simulink model "MCU_Stateflow_Analog"  (R2022b)
settings: Solver=FixedStepDiscrete  StartTime=0.0  StopTime=inf  FixedStep=0.002  RelTol=1e-3
undefined symbols (not defined in the file): ANALOG, cAgeingMode, cCurrentLoopMode, cNoneMode, cParaRecogMode, cSingleBoardMode, cSpeedLoopMode, cTorqueLoopMode, cVvvfOpenMode, FAULT, POWER_ON, STANDBY, TESTBED, VEHICLE, WORKING
libraries: simulink x9, SignalEditorBlockLib x1
(part 2 of 4)

== system MCU_Stateflow_Analog/Task_2ms/Arbitration/Initial ==
  note: WorkCmd初始化
  note: 在POWERON、STANDBY和FAULT模式下ModeSelect选择为cNoneMode
  Action Port : ActionPort  ActionPortLabel=if(u1 == 1)
  Constant : Constant  Value=0  OutDataTypeStr=single
  Constant1 : Constant  Value=cNoneMode  VectorParams1D=off  OutDataTypeStr=uint16
  Constant2 : Constant  Value=0  OutDataTypeStr=uint16
  Constant3 : Constant  Value=cNoneMode  VectorParams1D=off  OutDataTypeStr=uint16
  WorkState_ModeSelect : Outport
  WorkCmd_RunCmd : Outport  Port=2
  WorkCmd_DischargeCmd : Outport  Port=3
  WorkCmd_TorqueCmd : Outport  Port=4
  WorkCmd_ModeCmd : Outport  Port=5
  WorkCmd_CurrentCmd : Outport  Port=6
  WorkCmd_FreqCmd : Outport  Port=7
  WorkCmd_IsdCmd : Outport  Port=8
  WorkCmd_IsqCmd : Outport  Port=9
  WorkCmd_SpeedCmd : Outport  Port=10
  WorkCmd_ThetaCmd : Outport  Port=11
  wires:
  Constant/1 -> WorkCmd_TorqueCmd/1, WorkCmd_CurrentCmd/1, WorkCmd_FreqCmd/1, WorkCmd_ThetaCmd/1, WorkCmd_SpeedCmd/1, WorkCmd_IsqCmd/1, WorkCmd_IsdCmd/1
  Constant1/1 -> WorkState_ModeSelect/1
  Constant2/1 -> WorkCmd_RunCmd/1, WorkCmd_DischargeCmd/1
  Constant3/1 -> WorkCmd_ModeCmd/1

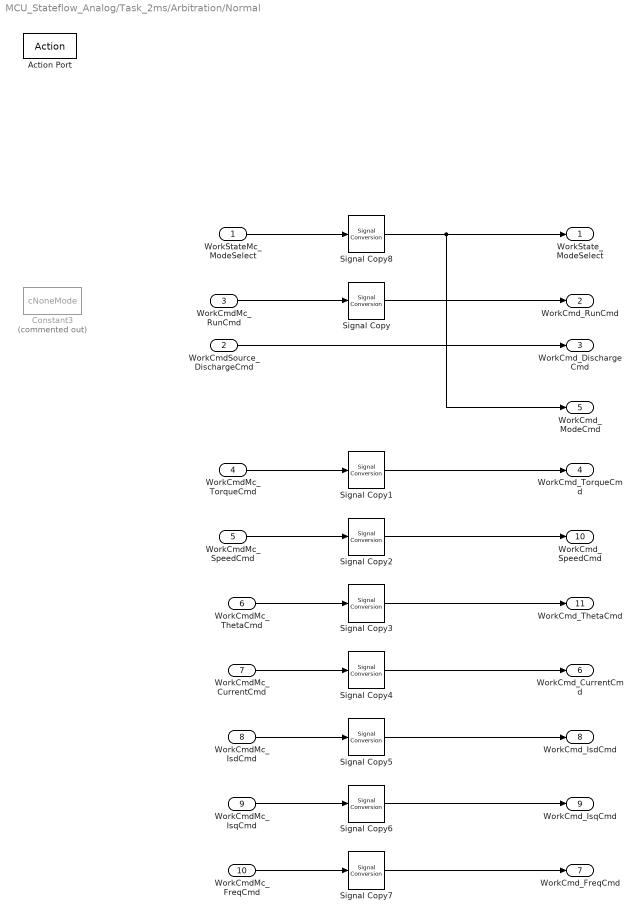
== system MCU_Stateflow_Analog/Task_2ms/Arbitration/Normal ==
  WorkStateMc_ModeSelect : Inport
  WorkCmdSource_DischargeCmd : Inport  Port=2
  WorkCmdMc_RunCmd : Inport  Port=3
  WorkCmdMc_TorqueCmd : Inport  Port=4
  WorkCmdMc_SpeedCmd : Inport  Port=5
  WorkCmdMc_ThetaCmd : Inport  Port=6
  WorkCmdMc_CurrentCmd : Inport  Port=7
  WorkCmdMc_IsdCmd : Inport  Port=8
  WorkCmdMc_IsqCmd : Inport  Port=9
  WorkCmdMc_FreqCmd : Inport  Port=10
  Action Port : ActionPort  ActionPortLabel=else
  Constant3 : Constant  Commented=on  Value=cNoneMode  VectorParams1D=off  OutDataTypeStr=uint16
  Signal Copy{,1..8} (9 alike) : SignalConversion  OverrideOpt=off
  WorkState_ModeSelect : Outport
  WorkCmd_RunCmd : Outport  Port=2
  WorkCmd_DischargeCmd : Outport  Port=3
  WorkCmd_TorqueCmd : Outport  Port=4
  WorkCmd_ModeCmd : Outport  Port=5
  WorkCmd_CurrentCmd : Outport  Port=6
  WorkCmd_FreqCmd : Outport  Port=7
  WorkCmd_IsdCmd : Outport  Port=8
  WorkCmd_IsqCmd : Outport  Port=9
  WorkCmd_SpeedCmd : Outport  Port=10
  WorkCmd_ThetaCmd : Outport  Port=11
  wires:
  WorkCmdMc_RunCmd/1 -> Signal Copy/1
  WorkCmdMc_TorqueCmd/1 -> Signal Copy1/1
  WorkCmdMc_SpeedCmd/1 -> Signal Copy2/1
  WorkCmdMc_ThetaCmd/1 -> Signal Copy3/1
  WorkCmdMc_CurrentCmd/1 -> Signal Copy4/1
  WorkCmdMc_IsdCmd/1 -> Signal Copy5/1
  WorkCmdMc_IsqCmd/1 -> Signal Copy6/1
  WorkCmdMc_FreqCmd/1 -> Signal Copy7/1
  WorkStateMc_ModeSelect/1 -> Signal Copy8/1
  Signal Copy8/1 -> WorkCmd_ModeCmd/1, WorkState_ModeSelect/1
  Signal Copy/1 -> WorkCmd_RunCmd/1
  Signal Copy1/1 -> WorkCmd_TorqueCmd/1
  Signal Copy2/1 -> WorkCmd_SpeedCmd/1
  Signal Copy3/1 -> WorkCmd_ThetaCmd/1
  Signal Copy4/1 -> WorkCmd_CurrentCmd/1
  Signal Copy5/1 -> WorkCmd_IsdCmd/1
  Signal Copy6/1 -> WorkCmd_IsqCmd/1
  Signal Copy7/1 -> WorkCmd_FreqCmd/1
  WorkCmdSource_DischargeCmd/1 -> WorkCmd_DischargeCmd/1

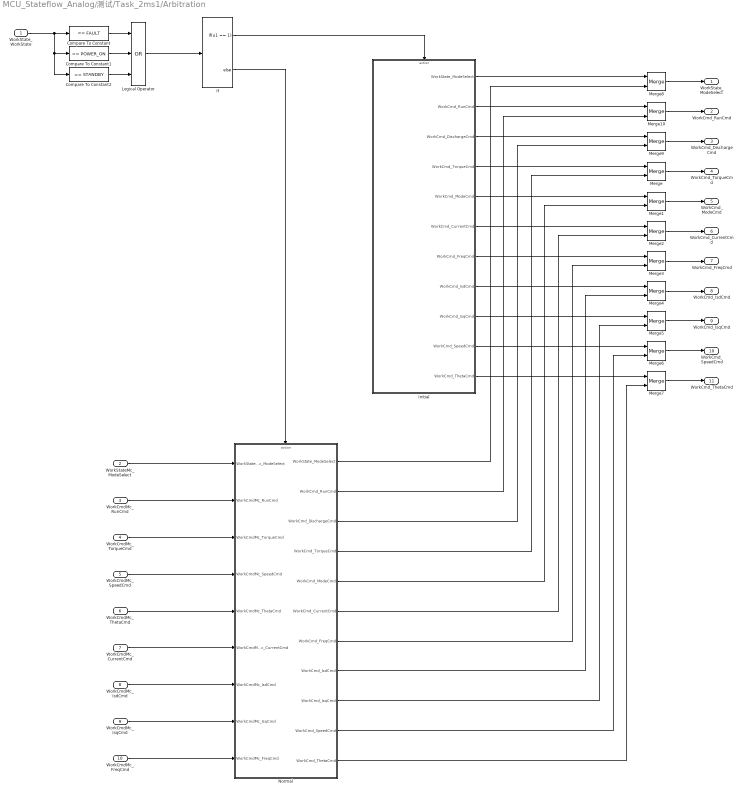
== system MCU_Stateflow_Analog/测试/Task_2ms1/Arbitration ==
  WorkState_WorkState : Inport
  WorkStateMc_ModeSelect : Inport  Port=2
  WorkCmdMc_RunCmd : Inport  Port=3
  WorkCmdMc_TorqueCmd : Inport  Port=4
  WorkCmdMc_SpeedCmd : Inport  Port=5
  WorkCmdMc_ThetaCmd : Inport  Port=6
  WorkCmdMc_CurrentCmd : Inport  Port=7
  WorkCmdMc_IsdCmd : Inport  Port=8
  WorkCmdMc_IsqCmd : Inport  Port=9
  WorkCmdMc_FreqCmd : Inport  Port=10
  Compare To Constant : simulink/Logic and Bit Operations/Compare To Constant  relop===  const=FAULT  OutDataTypeStr=boolean
  Compare To Constant1 : simulink/Logic and Bit Operations/Compare To Constant  relop===  const=POWER_ON  OutDataTypeStr=boolean
  Compare To Constant2 : simulink/Logic and Bit Operations/Compare To Constant  relop===  const=STANDBY  OutDataTypeStr=boolean
  If : If  IfExpression=u1 == 1
  Initial : Subsystem  TreatAsAtomicUnit=on
  Logical Operator : Logic  Operator=OR  Inputs=3  AllPortsSameDT=off  OutDataTypeStr=boolean
  Merge{,1..10} (11 alike) : Merge
  Normal : Subsystem  TreatAsAtomicUnit=on
  WorkState_ModeSelect : Outport
  WorkCmd_RunCmd : Outport  Port=2
  WorkCmd_DischargeCmd : Outport  Port=3
  WorkCmd_TorqueCmd : Outport  Port=4
  WorkCmd_ModeCmd : Outport  Port=5
  WorkCmd_CurrentCmd : Outport  Port=6
  WorkCmd_FreqCmd : Outport  Port=7
  WorkCmd_IsdCmd : Outport  Port=8
  WorkCmd_IsqCmd : Outport  Port=9
  WorkCmd_SpeedCmd : Outport  Port=10
  WorkCmd_ThetaCmd : Outport  Port=11
  wires:
  WorkState_WorkState/1 -> Compare To Constant2/1, Compare To Constant1/1, Compare To Constant/1
  Compare To Constant/1 -> Logical Operator/1
  Compare To Constant1/1 -> Logical Operator/2
  Compare To Constant2/1 -> Logical Operator/3
  Logical Operator/1 -> If/1
  If/1 -> Initial/Action
  If/2 -> Normal/Action
  Initial/11(WorkCmd_ThetaCmd) -> Merge7/1
  Initial/10(WorkCmd_SpeedCmd) -> Merge6/1
  Initial/9(WorkCmd_IsqCmd) -> Merge5/1
  Initial/8(WorkCmd_IsdCmd) -> Merge4/1
  Initial/7(WorkCmd_FreqCmd) -> Merge3/1
  Initial/6(WorkCmd_CurrentCmd) -> Merge2/1
  Initial/5(WorkCmd_ModeCmd) -> Merge1/1
  Initial/4(WorkCmd_TorqueCmd) -> Merge/1
  Initial/3(WorkCmd_DischargeCmd) -> Merge9/1
  WorkStateMc_ModeSelect/1 -> Normal/1(WorkStateMc_ModeSelect)
  WorkCmdMc_RunCmd/1 -> Normal/2(WorkCmdMc_RunCmd)
  WorkCmdMc_TorqueCmd/1 -> Normal/3(WorkCmdMc_TorqueCmd)
  WorkCmdMc_SpeedCmd/1 -> Normal/4(WorkCmdMc_SpeedCmd)
  WorkCmdMc_ThetaCmd/1 -> Normal/5(WorkCmdMc_ThetaCmd)
  WorkCmdMc_CurrentCmd/1 -> Normal/6(WorkCmdMc_CurrentCmd)
  WorkCmdMc_IsdCmd/1 -> Normal/7(WorkCmdMc_IsdCmd)
  WorkCmdMc_IsqCmd/1 -> Normal/8(WorkCmdMc_IsqCmd)
  WorkCmdMc_FreqCmd/1 -> Normal/9(WorkCmdMc_FreqCmd)
  Merge/1 -> WorkCmd_TorqueCmd/1
  Merge1/1 -> WorkCmd_ModeCmd/1
  Merge2/1 -> WorkCmd_CurrentCmd/1
  Merge3/1 -> WorkCmd_FreqCmd/1
  Merge4/1 -> WorkCmd_IsdCmd/1
  Merge5/1 -> WorkCmd_IsqCmd/1
  Merge6/1 -> WorkCmd_SpeedCmd/1
  Merge7/1 -> WorkCmd_ThetaCmd/1
  Initial/1(WorkState_ModeSelect) -> Merge8/1
  Merge8/1 -> WorkState_ModeSelect/1
  Initial/2(WorkCmd_RunCmd) -> Merge10/1
  Merge10/1 -> WorkCmd_RunCmd/1
  Merge9/1 -> WorkCmd_DischargeCmd/1
  Normal/1(WorkState_ModeSelect) -> Merge8/2
  Normal/2(WorkCmd_RunCmd) -> Merge10/2
  Normal/3(WorkCmd_DischargeCmd) -> Merge9/2
  Normal/4(WorkCmd_TorqueCmd) -> Merge/2
  Normal/5(WorkCmd_ModeCmd) -> Merge1/2
  Normal/6(WorkCmd_CurrentCmd) -> Merge2/2
  Normal/7(WorkCmd_FreqCmd) -> Merge3/2
  Normal/8(WorkCmd_IsdCmd) -> Merge4/2
  Normal/9(WorkCmd_IsqCmd) -> Merge5/2
  Normal/10(WorkCmd_SpeedCmd) -> Merge6/2
  Normal/11(WorkCmd_ThetaCmd) -> Merge7/2

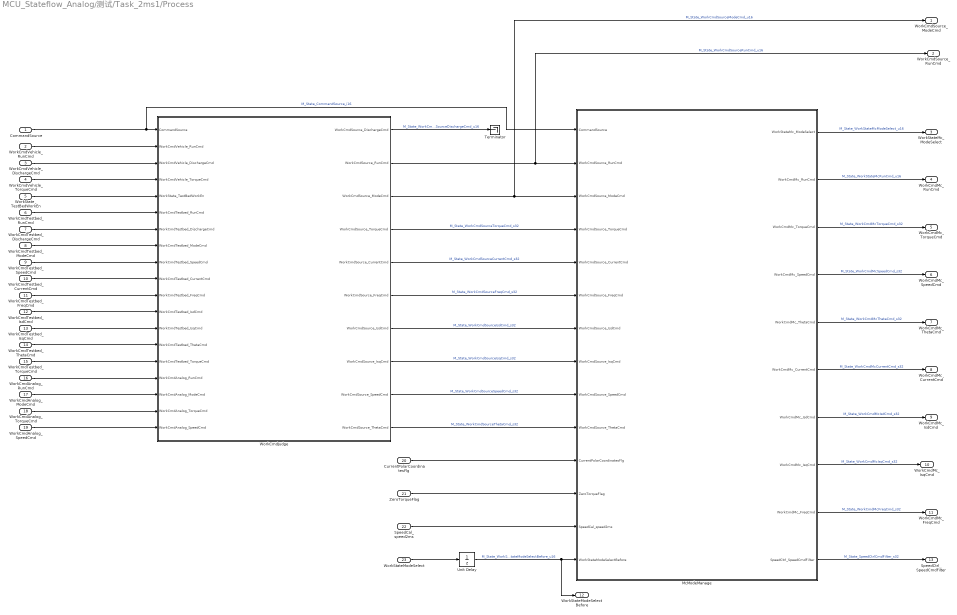
== system MCU_Stateflow_Analog/测试/Task_2ms1/Process ==
  CommandSource : Inport
  WorkCmdVehicle_RunCmd : Inport  Port=2
  WorkCmdVehicle_DischargeCmd : Inport  Port=3
  WorkCmdVehicle_TorqueCmd : Inport  Port=4
  WorkState_TestBedWorkEn : Inport  Port=5
  WorkCmdTestbed_RunCmd : Inport  Port=6
  WorkCmdTestbed_DischargeCmd : Inport  Port=7
  WorkCmdTestbed_ModeCmd : Inport  Port=8
  WorkCmdTestbed_SpeedCmd : Inport  Port=9
  WorkCmdTestbed_CurrentCmd : Inport  Port=10
  WorkCmdTestbed_FreqCmd : Inport  Port=11
  WorkCmdTestbed_IsdCmd : Inport  Port=12
  WorkCmdTestbed_IsqCmd : Inport  Port=13
  WorkCmdTestbed_ThetaCmd : Inport  Port=14
  WorkCmdTestbed_TorqueCmd : Inport  Port=15
  WorkCmdAnalog_RunCmd : Inport  Port=16
  WorkCmdAnalog_ModeCmd : Inport  Port=17
  WorkCmdAnalog_TorqueCmd : Inport  Port=18
  WorkCmdAnalog_SpeedCmd : Inport  Port=19
  CurrentPolarCoordinatesFlg : Inport  Port=20
  ZeroTorqueFlag : Inport  Port=21
  SpeedCal_speed2ms : Inport  Port=22
  WorkStateModeSelect : Inport  Port=23
  McModeManage : Stateflow chart  TreatAsAtomicUnit=on
      settings: RTWSystemCode=Nonreusable function  PortSchema="{\"entries\":[{\"content\":{\"sides\":[{\"content\":{\"connectorIds\":[\"In2\",\"In4\",\"In3\",\"In5\",\"In6\",\"In7\",\"In8\",\"In9\",\"In10\",\"In1\",\"In11\",\"In12\",\"In13\",\"In14\"]},\"type\":\"ConnectorPlacement.EquallySpacedRectSide\",\"uuid\":\"2e7d3842-0a61-4590-9292-7a5bc1b6d63e\"},{\"content\":{\"connectorIds\":[\"Out1\",\"Out2\",\"Out3\",\"Out4\",\"Out5\",\"Out6\",\"Out7\",\"Out8\",\"Out9\",\"Out10\"],\"side\":\"RIGHT\"},\"type\":\"ConnectorPlacement.EquallySpacedRectSide\",\"uuid\":\"fb66f02a-321f-47a6-a489-4b94442e22c8\"},{\"content\":{\"connectorIds\":[],\"side\":\"TOP\"},\"type\":\"ConnectorPlacement.EquallySpacedRectSide\",\"uuid\":\"26cfdcf8-827e-48d9-aa42-40739db869be\"},{\"content\":{\"connectorIds\":[],\"side\":\"BOTTOM\"},\"type\":\"ConnectorPlacement.EquallySpacedRectSide\",\"uuid\":\"3bc2be8d-756f-48d1-976e-919451ea6fa2\"}]},\"type\":\"ConnectorPlacement.EquallySpacedConnector\",\"uuid\":\"eb156a25-beb1-4594-a414-e9203ec852c3\"}],\"packageUris\":[\"http://schema.mathworks.com/mf0/Connector/R2020b\"],\"version\":\"1.0\"}"
  Terminator : Terminator
  Unit Delay : UnitDelay  SampleTime=-1  HasFrameUpgradeWarning=on
  WorkCmdJudge : Stateflow chart  TreatAsAtomicUnit=on
      settings: RTWSystemCode=Nonreusable function  PortSchema="{\"entries\":[{\"content\":{\"sides\":[{\"content\":{\"connectorIds\":[\"In2\",\"In3\",\"In4\",\"In15\",\"In5\",\"In6\",\"In7\",\"In8\",\"In9\",\"In10\",\"In11\",\"In12\",\"In13\",\"In14\",\"In16\",\"In17\",\"In1\",\"In19\",\"In18\"]},\"type\":\"ConnectorPlacement.EquallySpacedRectSide\",\"uuid\":\"08f79912-2405-4f04-9254-689ee53f44b9\"},{\"content\":{\"connectorIds\":[\"Out1\",\"Out2\",\"Out3\",\"Out10\",\"Out4\",\"Out5\",\"Out6\",\"Out7\",\"Out8\",\"Out9\"],\"side\":\"RIGHT\"},\"type\":\"ConnectorPlacement.EquallySpacedRectSide\",\"uuid\":\"8406ee0b-fe03-429b-8d11-a315759dccf9\"},{\"content\":{\"connectorIds\":[],\"side\":\"TOP\"},\"type\":\"ConnectorPlacement.EquallySpacedRectSide\",\"uuid\":\"82a87416-6ee6-4a7e-925f-181c5fe86ae8\"},{\"content\":{\"connectorIds\":[],\"side\":\"BOTTOM\"},\"type\":\"ConnectorPlacement.EquallySpacedRectSide\",\"uuid\":\"850ffd8e-4d4e-428c-999d-6858cee77358\"}]},\"type\":\"ConnectorPlacement.EquallySpacedConnector\",\"uuid\":\"ba5e9ad6-4f64-4c0c-82e6-bf977e3fd6e6\"}],\"packageUris\":[\"http://schema.mathworks.com/mf0/Connector/R2020b\"],\"version\":\"1.0\"}"
  WorkCmdSource_ModeCmd : Outport
  WorkCmdSource_RunCmd : Outport  Port=2
  WorkStateMc_ModeSelect : Outport  Port=3
  WorkCmdMc_RunCmd : Outport  Port=4
  WorkCmdMc_TorqueCmd : Outport  Port=5
  WorkCmdMc_SpeedCmd : Outport  Port=6
  WorkCmdMc_ThetaCmd : Outport  Port=7
  WorkCmdMc_CurrentCmd : Outport  Port=8
  WorkCmdMc_IsdCmd : Outport  Port=9
  WorkCmdMc_IsqCmd : Outport  Port=10
  WorkCmdMc_FreqCmd : Outport  Port=11
  WorkStateModeSelectBefore : Outport  Port=12
  SpeedCtrl_SpeedCmdFilter : Outport  Port=13
  wires:
  WorkCmdJudge/8(WorkCmdSource_SpeedCmd) -> McModeManage/10(WorkCmdSource_SpeedCmd)  "M_State_WorkCmdSourceSpeedCmd_s32"
  CommandSource/1 -> WorkCmdJudge/2(CommandSource), McModeManage/2(CommandSource)  "M_State_CommandSource_i16"
  WorkCmdJudge/4(WorkCmdSource_CurrentCmd) -> McModeManage/6(WorkCmdSource_CurrentCmd)  "M_State_WorkCmdSourceCurrentCmd_s32"
  WorkCmdJudge/6(WorkCmdSource_IsdCmd) -> McModeManage/8(WorkCmdSource_IsdCmd)  "M_State_WorkCmdSourceIsdCmd_s32"
  WorkCmdJudge/2(WorkCmdSource_RunCmd) -> WorkCmdSource_RunCmd/1, McModeManage/4(WorkCmdSource_RunCmd)  "M_State_WorkCmdSourceRunCmd_u16"
  WorkCmdTestbed_ThetaCmd/1 -> WorkCmdJudge/14(WorkCmdTestbed_ThetaCmd)
  WorkCmdJudge/7(WorkCmdSource_IsqCmd) -> McModeManage/9(WorkCmdSource_IsqCmd)  "M_State_WorkCmdSourceIsqCmd_s32"
  McModeManage/9(WorkCmdMc_FreqCmd) -> WorkCmdMc_FreqCmd/1  "M_State_WorkCmdMcFreqCmd_s32"
  McModeManage/2(WorkCmdMc_RunCmd) -> WorkCmdMc_RunCmd/1  "M_State_WorkStateMcRunCmd_u16"
  WorkCmdJudge/5(WorkCmdSource_FreqCmd) -> McModeManage/7(WorkCmdSource_FreqCmd)  "M_State_WorkCmdSourceFreqCmd_s32"
  WorkCmdJudge/10(WorkCmdSource_TorqueCmd) -> McModeManage/5(WorkCmdSource_TorqueCmd)  "M_State_WorkCmdSourceTorqueCmd_s32"
  McModeManage/4(WorkCmdMc_SpeedCmd) -> WorkCmdMc_SpeedCmd/1  "M_State_WorkCmdMcSpeedCmd_s32"
  WorkCmdJudge/9(WorkCmdSource_ThetaCmd) -> McModeManage/1(WorkCmdSource_ThetaCmd)  "M_State_WorkCmdSourceThetaCmd_s32"
  WorkCmdVehicle_RunCmd/1 -> WorkCmdJudge/3(WorkCmdVehicle_RunCmd)
  WorkCmdTestbed_IsdCmd/1 -> WorkCmdJudge/12(WorkCmdTestbed_IsdCmd)
  WorkCmdTestbed_IsqCmd/1 -> WorkCmdJudge/13(WorkCmdTestbed_IsqCmd)
  WorkCmdJudge/1(WorkCmdSource_DischargeCmd) -> Terminator/1  "M_State_WorkCmdSourceDischargeCmd_u16"
  McModeManage/1(WorkStateMc_ModeSelect) -> WorkStateMc_ModeSelect/1  "M_State_WorkStateMcModeSelect_u16"
  WorkCmdTestbed_TorqueCmd/1 -> WorkCmdJudge/16(WorkCmdTestbed_TorqueCmd)
  WorkCmdJudge/3(WorkCmdSource_ModeCmd) -> WorkCmdSource_ModeCmd/1, McModeManage/3(WorkCmdSource_ModeCmd)  "M_State_WorkCmdSourceModeCmd_u16"
  WorkCmdTestbed_ModeCmd/1 -> WorkCmdJudge/8(WorkCmdTestbed_ModeCmd)
  WorkCmdTestbed_DischargeCmd/1 -> WorkCmdJudge/7(WorkCmdTestbed_DischargeCmd)
  WorkCmdTestbed_RunCmd/1 -> WorkCmdJudge/6(WorkCmdTestbed_RunCmd)
  WorkCmdVehicle_DischargeCmd/1 -> WorkCmdJudge/4(WorkCmdVehicle_DischargeCmd)
  WorkCmdVehicle_TorqueCmd/1 -> WorkCmdJudge/15(WorkCmdVehicle_TorqueCmd)
  WorkState_TestBedWorkEn/1 -> WorkCmdJudge/5(WorkState_TestBedWorkEn)
  WorkCmdTestbed_CurrentCmd/1 -> WorkCmdJudge/10(WorkCmdTestbed_CurrentCmd)
  McModeManage/6(WorkCmdMc_CurrentCmd) -> WorkCmdMc_CurrentCmd/1  "M_State_WorkCmdMcCurrentCmd_s32"
  McModeManage/5(WorkCmdMc_ThetaCmd) -> WorkCmdMc_ThetaCmd/1  "M_State_WorkCmdMcThetaCmd_s32"
  McModeManage/7(WorkCmdMc_IsdCmd) -> WorkCmdMc_IsdCmd/1  "M_State_WorkCmdMcIsdCmd_s32"
  WorkCmdTestbed_SpeedCmd/1 -> WorkCmdJudge/9(WorkCmdTestbed_SpeedCmd)
  McModeManage/3(WorkCmdMc_TorqueCmd) -> WorkCmdMc_TorqueCmd/1  "M_State_WorkCmdMcTorqueCmd_s32"
  McModeManage/8(WorkCmdMc_IsqCmd) -> WorkCmdMc_IsqCmd/1  "M_State_WorkCmdMcIsqCmd_s32"
  WorkCmdTestbed_FreqCmd/1 -> WorkCmdJudge/11(WorkCmdTestbed_FreqCmd)
  WorkStateModeSelect/1 -> Unit Delay/1
  Unit Delay/1 -> McModeManage/14(WorkStateModeSelectBefore), WorkStateModeSelectBefore/1  "M_State_WorkStateModeSelectBefore_u16"
  WorkCmdAnalog_RunCmd/1 -> WorkCmdJudge/17(WorkCmdAnalog_RunCmd)
  WorkCmdAnalog_ModeCmd/1 -> WorkCmdJudge/1(WorkCmdAnalog_ModeCmd)
  WorkCmdAnalog_TorqueCmd/1 -> WorkCmdJudge/19(WorkCmdAnalog_TorqueCmd)
  WorkCmdAnalog_SpeedCmd/1 -> WorkCmdJudge/18(WorkCmdAnalog_SpeedCmd)
  CurrentPolarCoordinatesFlg/1 -> McModeManage/11(CurrentPolarCoordinatesFlg)
  ZeroTorqueFlag/1 -> McModeManage/12(ZeroTorqueFlag)
  SpeedCal_speed2ms/1 -> McModeManage/13(SpeedCal_speed2ms)
  McModeManage/10(SpeedCtrl_SpeedCmdFilter) -> SpeedCtrl_SpeedCmdFilter/1  "M_State_SpeedCtrlCmdFilter_s32"

== system MCU_Stateflow_Analog/测试/Task_2ms1/草稿 ==
  Chart : Stateflow chart  Commented=on  TreatAsAtomicUnit=on
      settings: PortSchema="{\"entries\":[{\"content\":{\"sides\":[{\"content\":{\"connectorIds\":[\"In2\",\"In4\",\"In3\",\"In5\",\"In6\",\"In7\",\"In8\",\"In9\",\"In10\",\"In11\",\"In1\"]},\"type\":\"ConnectorPlacement.EquallySpacedRectSide\",\"uuid\":\"2e7d3842-0a61-4590-9292-7a5bc1b6d63e\"},{\"content\":{\"connectorIds\":[\"Out1\",\"Out2\",\"Out3\",\"Out4\",\"Out5\",\"Out6\",\"Out7\",\"Out8\",\"Out9\"],\"side\":\"RIGHT\"},\"type\":\"ConnectorPlacement.EquallySpacedRectSide\",\"uuid\":\"fb66f02a-321f-47a6-a489-4b94442e22c8\"},{\"content\":{\"connectorIds\":[],\"side\":\"TOP\"},\"type\":\"ConnectorPlacement.EquallySpacedRectSide\",\"uuid\":\"26cfdcf8-827e-48d9-aa42-40739db869be\"},{\"content\":{\"connectorIds\":[],\"side\":\"BOTTOM\"},\"type\":\"ConnectorPlacement.EquallySpacedRectSide\",\"uuid\":\"3bc2be8d-756f-48d1-976e-919451ea6fa2\"}]},\"type\":\"ConnectorPlacement.EquallySpacedConnector\",\"uuid\":\"eb156a25-beb1-4594-a414-e9203ec852c3\"}],\"packageUris\":[\"http://schema.mathworks.com/mf0/Connector/R2020b\"],\"version\":\"1.0\"}"
  Chart2 : Stateflow chart  Commented=on  TreatAsAtomicUnit=on
      settings: PortSchema="{\"entries\":[{\"content\":{\"sides\":[{\"content\":{\"connectorIds\":[\"In2\",\"In4\",\"In3\",\"In5\",\"In6\",\"In7\",\"In8\",\"In9\",\"In10\",\"In1\",\"In11\"]},\"type\":\"ConnectorPlacement.EquallySpacedRectSide\",\"uuid\":\"2e7d3842-0a61-4590-9292-7a5bc1b6d63e\"},{\"content\":{\"connectorIds\":[\"Out1\",\"Out2\",\"Out3\",\"Out4\",\"Out5\",\"Out6\",\"Out7\",\"Out8\",\"Out9\"],\"side\":\"RIGHT\"},\"type\":\"ConnectorPlacement.EquallySpacedRectSide\",\"uuid\":\"fb66f02a-321f-47a6-a489-4b94442e22c8\"},{\"content\":{\"connectorIds\":[],\"side\":\"TOP\"},\"type\":\"ConnectorPlacement.EquallySpacedRectSide\",\"uuid\":\"26cfdcf8-827e-48d9-aa42-40739db869be\"},{\"content\":{\"connectorIds\":[],\"side\":\"BOTTOM\"},\"type\":\"ConnectorPlacement.EquallySpacedRectSide\",\"uuid\":\"3bc2be8d-756f-48d1-976e-919451ea6fa2\"}]},\"type\":\"ConnectorPlacement.EquallySpacedConnector\",\"uuid\":\"eb156a25-beb1-4594-a414-e9203ec852c3\"}],\"packageUris\":[\"http://schema.mathworks.com/mf0/Connector/R2020b\"],\"version\":\"1.0\"}"
  MotorState1 : Stateflow chart  Commented=on  TreatAsAtomicUnit=on
  MotorState2 : Stateflow chart  Commented=on  TreatAsAtomicUnit=on
      settings: PortSchema="{\"entries\":[{\"content\":{\"sides\":[{\"content\":{\"connectorIds\":[\"In12\",\"In7\",\"In8\",\"In9\",\"In10\",\"In11\",\"In13\",\"In14\",\"In6\",\"In15\",\"In5\",\"In4\",\"In3\",\"In2\",\"In1\"]},\"type\":\"ConnectorPlacement.EquallySpacedRectSide\",\"uuid\":\"e0adab7d-9c82-44fd-b38c-331bb9d71454\"},{\"content\":{\"connectorIds\":[\"Out1\",\"Out2\",\"Out3\"],\"side\":\"RIGHT\"},\"type\":\"ConnectorPlacement.EquallySpacedRectSide\",\"uuid\":\"98ad1acc-debf-46f0-91aa-4bd2062f60b6\"},{\"content\":{\"connectorIds\":[],\"side\":\"TOP\"},\"type\":\"ConnectorPlacement.EquallySpacedRectSide\",\"uuid\":\"a7c2d312-245c-4ce1-bea5-1bac95c515f1\"},{\"content\":{\"connectorIds\":[],\"side\":\"BOTTOM\"},\"type\":\"ConnectorPlacement.EquallySpacedRectSide\",\"uuid\":\"175f3b6b-1019-4e6e-83d9-bf4c82f74bc8\"}]},\"type\":\"ConnectorPlacement.EquallySpacedConnector\",\"uuid\":\"df312d8c-c57e-4b1a-958b-330641c1b4d1\"}],\"packageUris\":[\"http://schema.mathworks.com/mf0/Connector/R2020b\"],\"version\":\"1.0\"}"
  MotorState3 : Stateflow chart  TreatAsAtomicUnit=on
      settings: PortSchema="{\"entries\":[{\"content\":{\"sides\":[{\"content\":{\"connectorIds\":[\"In5\",\"In1\",\"In2\",\"In3\",\"In4\"]},\"type\":\"ConnectorPlacement.EquallySpacedRectSide\",\"uuid\":\"e0adab7d-9c82-44fd-b38c-331bb9d71454\"},{\"content\":{\"connectorIds\":[\"Out1\",\"Out2\",\"Out3\"],\"side\":\"RIGHT\"},\"type\":\"ConnectorPlacement.EquallySpacedRectSide\",\"uuid\":\"98ad1acc-debf-46f0-91aa-4bd2062f60b6\"},{\"content\":{\"connectorIds\":[],\"side\":\"TOP\"},\"type\":\"ConnectorPlacement.EquallySpacedRectSide\",\"uuid\":\"a7c2d312-245c-4ce1-bea5-1bac95c515f1\"},{\"content\":{\"connectorIds\":[],\"side\":\"BOTTOM\"},\"type\":\"ConnectorPlacement.EquallySpacedRectSide\",\"uuid\":\"175f3b6b-1019-4e6e-83d9-bf4c82f74bc8\"}]},\"type\":\"ConnectorPlacement.EquallySpacedConnector\",\"uuid\":\"df312d8c-c57e-4b1a-958b-330641c1b4d1\"}],\"packageUris\":[\"http://schema.mathworks.com/mf0/Connector/R2020b\"],\"version\":\"1.0\"}"
  MotorState4 : Stateflow chart  Commented=on  TreatAsAtomicUnit=on
      settings: PortSchema="{\"entries\":[{\"content\":{\"sides\":[{\"content\":{\"connectorIds\":[\"In4\",\"In3\",\"In1\",\"In2\",\"In5\"]},\"type\":\"ConnectorPlacement.EquallySpacedRectSide\",\"uuid\":\"e0adab7d-9c82-44fd-b38c-331bb9d71454\"},{\"content\":{\"connectorIds\":[\"Out1\",\"Out2\",\"Out3\"],\"side\":\"RIGHT\"},\"type\":\"ConnectorPlacement.EquallySpacedRectSide\",\"uuid\":\"98ad1acc-debf-46f0-91aa-4bd2062f60b6\"},{\"content\":{\"connectorIds\":[],\"side\":\"TOP\"},\"type\":\"ConnectorPlacement.EquallySpacedRectSide\",\"uuid\":\"a7c2d312-245c-4ce1-bea5-1bac95c515f1\"},{\"content\":{\"connectorIds\":[],\"side\":\"BOTTOM\"},\"type\":\"ConnectorPlacement.EquallySpacedRectSide\",\"uuid\":\"175f3b6b-1019-4e6e-83d9-bf4c82f74bc8\"}]},\"type\":\"ConnectorPlacement.EquallySpacedConnector\",\"uuid\":\"df312d8c-c57e-4b1a-958b-330641c1b4d1\"}],\"packageUris\":[\"http://schema.mathworks.com/mf0/Connector/R2020b\"],\"version\":\"1.0\"}"

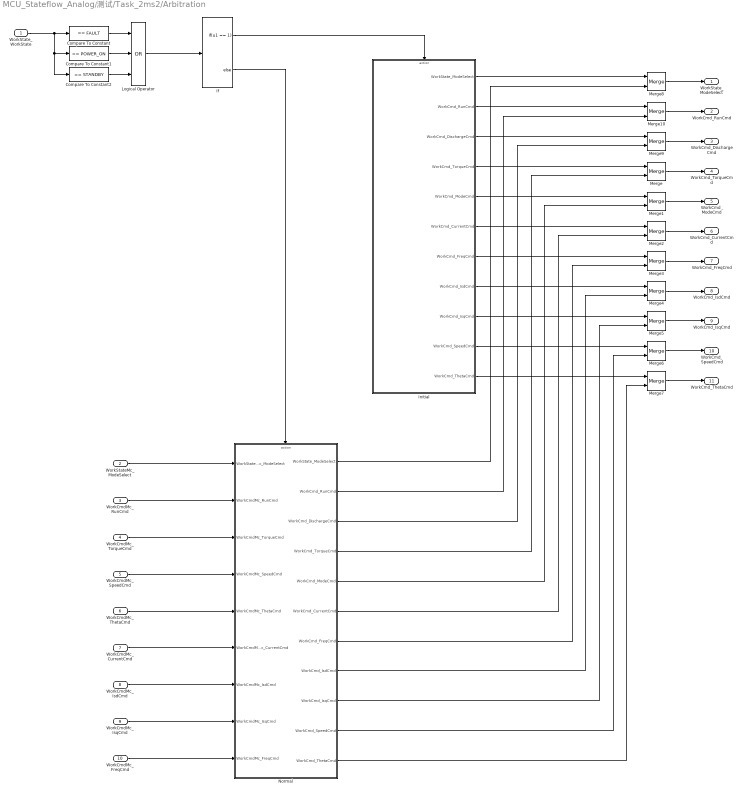
== system MCU_Stateflow_Analog/测试/Task_2ms2/Arbitration ==
  WorkState_WorkState : Inport
  WorkStateMc_ModeSelect : Inport  Port=2
  WorkCmdMc_RunCmd : Inport  Port=3
  WorkCmdMc_TorqueCmd : Inport  Port=4
  WorkCmdMc_SpeedCmd : Inport  Port=5
  WorkCmdMc_ThetaCmd : Inport  Port=6
  WorkCmdMc_CurrentCmd : Inport  Port=7
  WorkCmdMc_IsdCmd : Inport  Port=8
  WorkCmdMc_IsqCmd : Inport  Port=9
  WorkCmdMc_FreqCmd : Inport  Port=10
  Compare To Constant : simulink/Logic and Bit Operations/Compare To Constant  relop===  const=FAULT  OutDataTypeStr=boolean
  Compare To Constant1 : simulink/Logic and Bit Operations/Compare To Constant  relop===  const=POWER_ON  OutDataTypeStr=boolean
  Compare To Constant2 : simulink/Logic and Bit Operations/Compare To Constant  relop===  const=STANDBY  OutDataTypeStr=boolean
  If : If  IfExpression=u1 == 1
  Initial : Subsystem  TreatAsAtomicUnit=on
  Logical Operator : Logic  Operator=OR  Inputs=3  AllPortsSameDT=off  OutDataTypeStr=boolean
  Merge{,1..10} (11 alike) : Merge
  Normal : Subsystem  TreatAsAtomicUnit=on
  WorkState_ModeSelect : Outport
  WorkCmd_RunCmd : Outport  Port=2
  WorkCmd_DischargeCmd : Outport  Port=3
  WorkCmd_TorqueCmd : Outport  Port=4
  WorkCmd_ModeCmd : Outport  Port=5
  WorkCmd_CurrentCmd : Outport  Port=6
  WorkCmd_FreqCmd : Outport  Port=7
  WorkCmd_IsdCmd : Outport  Port=8
  WorkCmd_IsqCmd : Outport  Port=9
  WorkCmd_SpeedCmd : Outport  Port=10
  WorkCmd_ThetaCmd : Outport  Port=11
  wires:
  WorkState_WorkState/1 -> Compare To Constant2/1, Compare To Constant1/1, Compare To Constant/1
  Compare To Constant/1 -> Logical Operator/1
  Compare To Constant1/1 -> Logical Operator/2
  Compare To Constant2/1 -> Logical Operator/3
  Logical Operator/1 -> If/1
  If/1 -> Initial/Action
  If/2 -> Normal/Action
  Initial/11(WorkCmd_ThetaCmd) -> Merge7/1
  Initial/10(WorkCmd_SpeedCmd) -> Merge6/1
  Initial/9(WorkCmd_IsqCmd) -> Merge5/1
  Initial/8(WorkCmd_IsdCmd) -> Merge4/1
  Initial/7(WorkCmd_FreqCmd) -> Merge3/1
  Initial/6(WorkCmd_CurrentCmd) -> Merge2/1
  Initial/5(WorkCmd_ModeCmd) -> Merge1/1
  Initial/4(WorkCmd_TorqueCmd) -> Merge/1
  Initial/3(WorkCmd_DischargeCmd) -> Merge9/1
  WorkStateMc_ModeSelect/1 -> Normal/1(WorkStateMc_ModeSelect)
  WorkCmdMc_RunCmd/1 -> Normal/2(WorkCmdMc_RunCmd)
  WorkCmdMc_TorqueCmd/1 -> Normal/3(WorkCmdMc_TorqueCmd)
  WorkCmdMc_SpeedCmd/1 -> Normal/4(WorkCmdMc_SpeedCmd)
  WorkCmdMc_ThetaCmd/1 -> Normal/5(WorkCmdMc_ThetaCmd)
  WorkCmdMc_CurrentCmd/1 -> Normal/6(WorkCmdMc_CurrentCmd)
  WorkCmdMc_IsdCmd/1 -> Normal/7(WorkCmdMc_IsdCmd)
  WorkCmdMc_IsqCmd/1 -> Normal/8(WorkCmdMc_IsqCmd)
  WorkCmdMc_FreqCmd/1 -> Normal/9(WorkCmdMc_FreqCmd)
  Merge/1 -> WorkCmd_TorqueCmd/1
  Merge1/1 -> WorkCmd_ModeCmd/1
  Merge2/1 -> WorkCmd_CurrentCmd/1
  Merge3/1 -> WorkCmd_FreqCmd/1
  Merge4/1 -> WorkCmd_IsdCmd/1
  Merge5/1 -> WorkCmd_IsqCmd/1
  Merge6/1 -> WorkCmd_SpeedCmd/1
  Merge7/1 -> WorkCmd_ThetaCmd/1
  Initial/1(WorkState_ModeSelect) -> Merge8/1
  Merge8/1 -> WorkState_ModeSelect/1
  Initial/2(WorkCmd_RunCmd) -> Merge10/1
  Merge10/1 -> WorkCmd_RunCmd/1
  Merge9/1 -> WorkCmd_DischargeCmd/1
  Normal/1(WorkState_ModeSelect) -> Merge8/2
  Normal/2(WorkCmd_RunCmd) -> Merge10/2
  Normal/3(WorkCmd_DischargeCmd) -> Merge9/2
  Normal/4(WorkCmd_TorqueCmd) -> Merge/2
  Normal/5(WorkCmd_ModeCmd) -> Merge1/2
  Normal/6(WorkCmd_CurrentCmd) -> Merge2/2
  Normal/7(WorkCmd_FreqCmd) -> Merge3/2
  Normal/8(WorkCmd_IsdCmd) -> Merge4/2
  Normal/9(WorkCmd_IsqCmd) -> Merge5/2
  Normal/10(WorkCmd_SpeedCmd) -> Merge6/2
  Normal/11(WorkCmd_ThetaCmd) -> Merge7/2

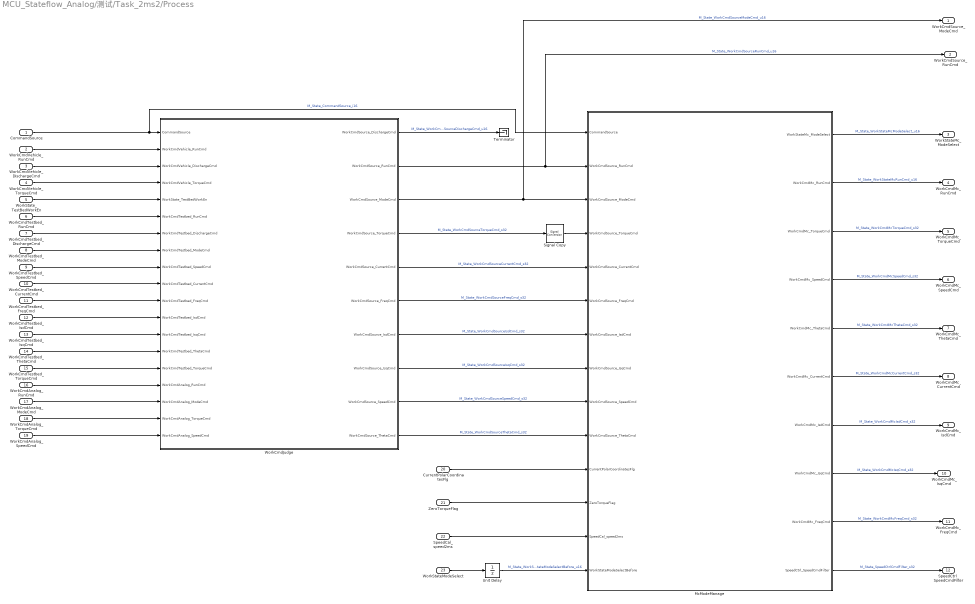
== system MCU_Stateflow_Analog/测试/Task_2ms2/Process ==
  CommandSource : Inport
  WorkCmdVehicle_RunCmd : Inport  Port=2
  WorkCmdVehicle_DischargeCmd : Inport  Port=3
  WorkCmdVehicle_TorqueCmd : Inport  Port=4
  WorkState_TestBedWorkEn : Inport  Port=5
  WorkCmdTestbed_RunCmd : Inport  Port=6
  WorkCmdTestbed_DischargeCmd : Inport  Port=7
  WorkCmdTestbed_ModeCmd : Inport  Port=8
  WorkCmdTestbed_SpeedCmd : Inport  Port=9
  WorkCmdTestbed_CurrentCmd : Inport  Port=10
  WorkCmdTestbed_FreqCmd : Inport  Port=11
  WorkCmdTestbed_IsdCmd : Inport  Port=12
  WorkCmdTestbed_IsqCmd : Inport  Port=13
  WorkCmdTestbed_ThetaCmd : Inport  Port=14
  WorkCmdTestbed_TorqueCmd : Inport  Port=15
  WorkCmdAnalog_RunCmd : Inport  Port=16
  WorkCmdAnalog_ModeCmd : Inport  Port=17
  WorkCmdAnalog_TorqueCmd : Inport  Port=18
  WorkCmdAnalog_SpeedCmd : Inport  Port=19
  CurrentPolarCoordinatesFlg : Inport  Port=20
  ZeroTorqueFlag : Inport  Port=21
  SpeedCal_speed2ms : Inport  Port=22
  WorkStateModeSelect : Inport  Port=23
  McModeManage : Stateflow chart  TreatAsAtomicUnit=on
      settings: RTWSystemCode=Reusable function  FunctionInterfaceSpec=Allow arguments (Optimized)  PortSchema="{\"entries\":[{\"content\":{\"sides\":[{\"content\":{\"connectorIds\":[\"In2\",\"In4\",\"In3\",\"In5\",\"In6\",\"In7\",\"In8\",\"In9\",\"In10\",\"In1\",\"In11\",\"In12\",\"In13\",\"In14\"]},\"type\":\"ConnectorPlacement.EquallySpacedRectSide\",\"uuid\":\"2e7d3842-0a61-4590-9292-7a5bc1b6d63e\"},{\"content\":{\"connectorIds\":[\"Out1\",\"Out2\",\"Out3\",\"Out4\",\"Out5\",\"Out6\",\"Out7\",\"Out8\",\"Out9\",\"Out10\"],\"side\":\"RIGHT\"},\"type\":\"ConnectorPlacement.EquallySpacedRectSide\",\"uuid\":\"fb66f02a-321f-47a6-a489-4b94442e22c8\"},{\"content\":{\"connectorIds\":[],\"side\":\"TOP\"},\"type\":\"ConnectorPlacement.EquallySpacedRectSide\",\"uuid\":\"26cfdcf8-827e-48d9-aa42-40739db869be\"},{\"content\":{\"connectorIds\":[],\"side\":\"BOTTOM\"},\"type\":\"ConnectorPlacement.EquallySpacedRectSide\",\"uuid\":\"3bc2be8d-756f-48d1-976e-919451ea6fa2\"}]},\"type\":\"ConnectorPlacement.EquallySpacedConnector\",\"uuid\":\"eb156a25-beb1-4594-a414-e9203ec852c3\"}],\"packageUris\":[\"http://schema.mathworks.com/mf0/Connector/R2020b\"],\"version\":\"1.0\"}"
  Signal Copy : SignalConversion  OverrideOpt=off
  Terminator : Terminator
  Unit Delay : UnitDelay  SampleTime=-1  HasFrameUpgradeWarning=on
  WorkCmdJudge : Stateflow chart  TreatAsAtomicUnit=on
      settings: RTWSystemCode=Reusable function  RTWFcnNameOpts=Use subsystem name  FunctionInterfaceSpec=Allow arguments (Optimized)  PortSchema="{\"entries\":[{\"content\":{\"sides\":[{\"content\":{\"connectorIds\":[\"In2\",\"In3\",\"In4\",\"In15\",\"In5\",\"In6\",\"In7\",\"In8\",\"In9\",\"In10\",\"In11\",\"In12\",\"In13\",\"In14\",\"In16\",\"In17\",\"In1\",\"In19\",\"In18\"]},\"type\":\"ConnectorPlacement.EquallySpacedRectSide\",\"uuid\":\"08f79912-2405-4f04-9254-689ee53f44b9\"},{\"content\":{\"connectorIds\":[\"Out1\",\"Out2\",\"Out3\",\"Out10\",\"Out4\",\"Out5\",\"Out6\",\"Out7\",\"Out8\",\"Out9\"],\"side\":\"RIGHT\"},\"type\":\"ConnectorPlacement.EquallySpacedRectSide\",\"uuid\":\"8406ee0b-fe03-429b-8d11-a315759dccf9\"},{\"content\":{\"connectorIds\":[],\"side\":\"TOP\"},\"type\":\"ConnectorPlacement.EquallySpacedRectSide\",\"uuid\":\"82a87416-6ee6-4a7e-925f-181c5fe86ae8\"},{\"content\":{\"connectorIds\":[],\"side\":\"BOTTOM\"},\"type\":\"ConnectorPlacement.EquallySpacedRectSide\",\"uuid\":\"850ffd8e-4d4e-428c-999d-6858cee77358\"}]},\"type\":\"ConnectorPlacement.EquallySpacedConnector\",\"uuid\":\"ba5e9ad6-4f64-4c0c-82e6-bf977e3fd6e6\"}],\"packageUris\":[\"http://schema.mathworks.com/mf0/Connector/R2020b\"],\"version\":\"1.0\"}"
  WorkCmdSource_ModeCmd : Outport
  WorkCmdSource_RunCmd : Outport  Port=2
  WorkStateMc_ModeSelect : Outport  Port=3
  WorkCmdMc_RunCmd : Outport  Port=4
  WorkCmdMc_TorqueCmd : Outport  Port=5
  WorkCmdMc_SpeedCmd : Outport  Port=6
  WorkCmdMc_ThetaCmd : Outport  Port=7
  WorkCmdMc_CurrentCmd : Outport  Port=8
  WorkCmdMc_IsdCmd : Outport  Port=9
  WorkCmdMc_IsqCmd : Outport  Port=10
  WorkCmdMc_FreqCmd : Outport  Port=11
  SpeedCtrl_SpeedCmdFilter : Outport  Port=12
  wires:
  WorkCmdJudge/8(WorkCmdSource_SpeedCmd) -> McModeManage/10(WorkCmdSource_SpeedCmd)  "M_State_WorkCmdSourceSpeedCmd_s32"
  CommandSource/1 -> WorkCmdJudge/2(CommandSource), McModeManage/2(CommandSource)  "M_State_CommandSource_i16"
  WorkCmdJudge/4(WorkCmdSource_CurrentCmd) -> McModeManage/6(WorkCmdSource_CurrentCmd)  "M_State_WorkCmdSourceCurrentCmd_s32"
  WorkCmdJudge/6(WorkCmdSource_IsdCmd) -> McModeManage/8(WorkCmdSource_IsdCmd)  "M_State_WorkCmdSourceIsdCmd_s32"
  WorkCmdJudge/2(WorkCmdSource_RunCmd) -> WorkCmdSource_RunCmd/1, McModeManage/4(WorkCmdSource_RunCmd)  "M_State_WorkCmdSourceRunCmd_u16"
  WorkCmdTestbed_ThetaCmd/1 -> WorkCmdJudge/14(WorkCmdTestbed_ThetaCmd)
  WorkCmdJudge/7(WorkCmdSource_IsqCmd) -> McModeManage/9(WorkCmdSource_IsqCmd)  "M_State_WorkCmdSourceIsqCmd_s32"
  McModeManage/9(WorkCmdMc_FreqCmd) -> WorkCmdMc_FreqCmd/1  "M_State_WorkCmdMcFreqCmd_s32"
  McModeManage/2(WorkCmdMc_RunCmd) -> WorkCmdMc_RunCmd/1  "M_State_WorkStateMcRunCmd_u16"
  WorkCmdJudge/5(WorkCmdSource_FreqCmd) -> McModeManage/7(WorkCmdSource_FreqCmd)  "M_State_WorkCmdSourceFreqCmd_s32"
  WorkCmdJudge/10(WorkCmdSource_TorqueCmd) -> Signal Copy/1  "M_State_WorkCmdSourceTorqueCmd_s32"
  McModeManage/4(WorkCmdMc_SpeedCmd) -> WorkCmdMc_SpeedCmd/1  "M_State_WorkCmdMcSpeedCmd_s32"
  WorkCmdJudge/9(WorkCmdSource_ThetaCmd) -> McModeManage/1(WorkCmdSource_ThetaCmd)  "M_State_WorkCmdSourceThetaCmd_s32"
  WorkCmdVehicle_RunCmd/1 -> WorkCmdJudge/3(WorkCmdVehicle_RunCmd)
  WorkCmdTestbed_IsdCmd/1 -> WorkCmdJudge/12(WorkCmdTestbed_IsdCmd)
  WorkCmdTestbed_IsqCmd/1 -> WorkCmdJudge/13(WorkCmdTestbed_IsqCmd)
  WorkCmdJudge/1(WorkCmdSource_DischargeCmd) -> Terminator/1  "M_State_WorkCmdSourceDischargeCmd_u16"
  McModeManage/1(WorkStateMc_ModeSelect) -> WorkStateMc_ModeSelect/1  "M_State_WorkStateMcModeSelect_u16"
  WorkCmdTestbed_TorqueCmd/1 -> WorkCmdJudge/16(WorkCmdTestbed_TorqueCmd)
  WorkCmdJudge/3(WorkCmdSource_ModeCmd) -> WorkCmdSource_ModeCmd/1, McModeManage/3(WorkCmdSource_ModeCmd)  "M_State_WorkCmdSourceModeCmd_u16"
  WorkCmdTestbed_ModeCmd/1 -> WorkCmdJudge/8(WorkCmdTestbed_ModeCmd)
  WorkCmdTestbed_DischargeCmd/1 -> WorkCmdJudge/7(WorkCmdTestbed_DischargeCmd)
  WorkCmdTestbed_RunCmd/1 -> WorkCmdJudge/6(WorkCmdTestbed_RunCmd)
  WorkCmdVehicle_DischargeCmd/1 -> WorkCmdJudge/4(WorkCmdVehicle_DischargeCmd)
  WorkCmdVehicle_TorqueCmd/1 -> WorkCmdJudge/15(WorkCmdVehicle_TorqueCmd)
  WorkState_TestBedWorkEn/1 -> WorkCmdJudge/5(WorkState_TestBedWorkEn)
  WorkCmdTestbed_CurrentCmd/1 -> WorkCmdJudge/10(WorkCmdTestbed_CurrentCmd)
  McModeManage/6(WorkCmdMc_CurrentCmd) -> WorkCmdMc_CurrentCmd/1  "M_State_WorkCmdMcCurrentCmd_s32"
  McModeManage/5(WorkCmdMc_ThetaCmd) -> WorkCmdMc_ThetaCmd/1  "M_State_WorkCmdMcThetaCmd_s32"
  McModeManage/7(WorkCmdMc_IsdCmd) -> WorkCmdMc_IsdCmd/1  "M_State_WorkCmdMcIsdCmd_s32"
  WorkCmdTestbed_SpeedCmd/1 -> WorkCmdJudge/9(WorkCmdTestbed_SpeedCmd)
  McModeManage/3(WorkCmdMc_TorqueCmd) -> WorkCmdMc_TorqueCmd/1  "M_State_WorkCmdMcTorqueCmd_s32"
  McModeManage/8(WorkCmdMc_IsqCmd) -> WorkCmdMc_IsqCmd/1  "M_State_WorkCmdMcIsqCmd_s32"
  WorkCmdTestbed_FreqCmd/1 -> WorkCmdJudge/11(WorkCmdTestbed_FreqCmd)
  WorkStateModeSelect/1 -> Unit Delay/1
  Unit Delay/1 -> McModeManage/14(WorkStateModeSelectBefore)  "M_State_WorkStateModeSelectBefore_u16"
  WorkCmdAnalog_RunCmd/1 -> WorkCmdJudge/17(WorkCmdAnalog_RunCmd)
  WorkCmdAnalog_ModeCmd/1 -> WorkCmdJudge/1(WorkCmdAnalog_ModeCmd)
  WorkCmdAnalog_TorqueCmd/1 -> WorkCmdJudge/19(WorkCmdAnalog_TorqueCmd)
  WorkCmdAnalog_SpeedCmd/1 -> WorkCmdJudge/18(WorkCmdAnalog_SpeedCmd)
  CurrentPolarCoordinatesFlg/1 -> McModeManage/11(CurrentPolarCoordinatesFlg)
  ZeroTorqueFlag/1 -> McModeManage/12(ZeroTorqueFlag)
  SpeedCal_speed2ms/1 -> McModeManage/13(SpeedCal_speed2ms)
  McModeManage/10(SpeedCtrl_SpeedCmdFilter) -> SpeedCtrl_SpeedCmdFilter/1  "M_State_SpeedCtrlCmdFilter_s32"
  Signal Copy/1 -> McModeManage/5(WorkCmdSource_TorqueCmd)

== system MCU_Stateflow_Analog/测试/Task_2ms2/草稿 ==
  Chart : Stateflow chart  Commented=on  TreatAsAtomicUnit=on
      settings: PortSchema="{\"entries\":[{\"content\":{\"sides\":[{\"content\":{\"connectorIds\":[\"In2\",\"In4\",\"In3\",\"In5\",\"In6\",\"In7\",\"In8\",\"In9\",\"In10\",\"In11\",\"In1\"]},\"type\":\"ConnectorPlacement.EquallySpacedRectSide\",\"uuid\":\"2e7d3842-0a61-4590-9292-7a5bc1b6d63e\"},{\"content\":{\"connectorIds\":[\"Out1\",\"Out2\",\"Out3\",\"Out4\",\"Out5\",\"Out6\",\"Out7\",\"Out8\",\"Out9\"],\"side\":\"RIGHT\"},\"type\":\"ConnectorPlacement.EquallySpacedRectSide\",\"uuid\":\"fb66f02a-321f-47a6-a489-4b94442e22c8\"},{\"content\":{\"connectorIds\":[],\"side\":\"TOP\"},\"type\":\"ConnectorPlacement.EquallySpacedRectSide\",\"uuid\":\"26cfdcf8-827e-48d9-aa42-40739db869be\"},{\"content\":{\"connectorIds\":[],\"side\":\"BOTTOM\"},\"type\":\"ConnectorPlacement.EquallySpacedRectSide\",\"uuid\":\"3bc2be8d-756f-48d1-976e-919451ea6fa2\"}]},\"type\":\"ConnectorPlacement.EquallySpacedConnector\",\"uuid\":\"eb156a25-beb1-4594-a414-e9203ec852c3\"}],\"packageUris\":[\"http://schema.mathworks.com/mf0/Connector/R2020b\"],\"version\":\"1.0\"}"
  Chart2 : Stateflow chart  Commented=on  TreatAsAtomicUnit=on
      settings: PortSchema="{\"entries\":[{\"content\":{\"sides\":[{\"content\":{\"connectorIds\":[\"In2\",\"In4\",\"In3\",\"In5\",\"In6\",\"In7\",\"In8\",\"In9\",\"In10\",\"In1\",\"In11\"]},\"type\":\"ConnectorPlacement.EquallySpacedRectSide\",\"uuid\":\"2e7d3842-0a61-4590-9292-7a5bc1b6d63e\"},{\"content\":{\"connectorIds\":[\"Out1\",\"Out2\",\"Out3\",\"Out4\",\"Out5\",\"Out6\",\"Out7\",\"Out8\",\"Out9\"],\"side\":\"RIGHT\"},\"type\":\"ConnectorPlacement.EquallySpacedRectSide\",\"uuid\":\"fb66f02a-321f-47a6-a489-4b94442e22c8\"},{\"content\":{\"connectorIds\":[],\"side\":\"TOP\"},\"type\":\"ConnectorPlacement.EquallySpacedRectSide\",\"uuid\":\"26cfdcf8-827e-48d9-aa42-40739db869be\"},{\"content\":{\"connectorIds\":[],\"side\":\"BOTTOM\"},\"type\":\"ConnectorPlacement.EquallySpacedRectSide\",\"uuid\":\"3bc2be8d-756f-48d1-976e-919451ea6fa2\"}]},\"type\":\"ConnectorPlacement.EquallySpacedConnector\",\"uuid\":\"eb156a25-beb1-4594-a414-e9203ec852c3\"}],\"packageUris\":[\"http://schema.mathworks.com/mf0/Connector/R2020b\"],\"version\":\"1.0\"}"
  MotorState1 : Stateflow chart  Commented=on  TreatAsAtomicUnit=on
  MotorState2 : Stateflow chart  Commented=on  TreatAsAtomicUnit=on
      settings: PortSchema="{\"entries\":[{\"content\":{\"sides\":[{\"content\":{\"connectorIds\":[\"In12\",\"In7\",\"In8\",\"In9\",\"In10\",\"In11\",\"In13\",\"In14\",\"In6\",\"In15\",\"In5\",\"In4\",\"In3\",\"In2\",\"In1\"]},\"type\":\"ConnectorPlacement.EquallySpacedRectSide\",\"uuid\":\"e0adab7d-9c82-44fd-b38c-331bb9d71454\"},{\"content\":{\"connectorIds\":[\"Out1\",\"Out2\",\"Out3\"],\"side\":\"RIGHT\"},\"type\":\"ConnectorPlacement.EquallySpacedRectSide\",\"uuid\":\"98ad1acc-debf-46f0-91aa-4bd2062f60b6\"},{\"content\":{\"connectorIds\":[],\"side\":\"TOP\"},\"type\":\"ConnectorPlacement.EquallySpacedRectSide\",\"uuid\":\"a7c2d312-245c-4ce1-bea5-1bac95c515f1\"},{\"content\":{\"connectorIds\":[],\"side\":\"BOTTOM\"},\"type\":\"ConnectorPlacement.EquallySpacedRectSide\",\"uuid\":\"175f3b6b-1019-4e6e-83d9-bf4c82f74bc8\"}]},\"type\":\"ConnectorPlacement.EquallySpacedConnector\",\"uuid\":\"df312d8c-c57e-4b1a-958b-330641c1b4d1\"}],\"packageUris\":[\"http://schema.mathworks.com/mf0/Connector/R2020b\"],\"version\":\"1.0\"}"
  MotorState3 : Stateflow chart  TreatAsAtomicUnit=on
      settings: PortSchema="{\"entries\":[{\"content\":{\"sides\":[{\"content\":{\"connectorIds\":[\"In5\",\"In1\",\"In2\",\"In3\",\"In4\"]},\"type\":\"ConnectorPlacement.EquallySpacedRectSide\",\"uuid\":\"e0adab7d-9c82-44fd-b38c-331bb9d71454\"},{\"content\":{\"connectorIds\":[\"Out1\",\"Out2\",\"Out3\"],\"side\":\"RIGHT\"},\"type\":\"ConnectorPlacement.EquallySpacedRectSide\",\"uuid\":\"98ad1acc-debf-46f0-91aa-4bd2062f60b6\"},{\"content\":{\"connectorIds\":[],\"side\":\"TOP\"},\"type\":\"ConnectorPlacement.EquallySpacedRectSide\",\"uuid\":\"a7c2d312-245c-4ce1-bea5-1bac95c515f1\"},{\"content\":{\"connectorIds\":[],\"side\":\"BOTTOM\"},\"type\":\"ConnectorPlacement.EquallySpacedRectSide\",\"uuid\":\"175f3b6b-1019-4e6e-83d9-bf4c82f74bc8\"}]},\"type\":\"ConnectorPlacement.EquallySpacedConnector\",\"uuid\":\"df312d8c-c57e-4b1a-958b-330641c1b4d1\"}],\"packageUris\":[\"http://schema.mathworks.com/mf0/Connector/R2020b\"],\"version\":\"1.0\"}"
  MotorState4 : Stateflow chart  Commented=on  TreatAsAtomicUnit=on
      settings: PortSchema="{\"entries\":[{\"content\":{\"sides\":[{\"content\":{\"connectorIds\":[\"In4\",\"In3\",\"In1\",\"In2\",\"In5\"]},\"type\":\"ConnectorPlacement.EquallySpacedRectSide\",\"uuid\":\"e0adab7d-9c82-44fd-b38c-331bb9d71454\"},{\"content\":{\"connectorIds\":[\"Out1\",\"Out2\",\"Out3\"],\"side\":\"RIGHT\"},\"type\":\"ConnectorPlacement.EquallySpacedRectSide\",\"uuid\":\"98ad1acc-debf-46f0-91aa-4bd2062f60b6\"},{\"content\":{\"connectorIds\":[],\"side\":\"TOP\"},\"type\":\"ConnectorPlacement.EquallySpacedRectSide\",\"uuid\":\"a7c2d312-245c-4ce1-bea5-1bac95c515f1\"},{\"content\":{\"connectorIds\":[],\"side\":\"BOTTOM\"},\"type\":\"ConnectorPlacement.EquallySpacedRectSide\",\"uuid\":\"175f3b6b-1019-4e6e-83d9-bf4c82f74bc8\"}]},\"type\":\"ConnectorPlacement.EquallySpacedConnector\",\"uuid\":\"df312d8c-c57e-4b1a-958b-330641c1b4d1\"}],\"packageUris\":[\"http://schema.mathworks.com/mf0/Connector/R2020b\"],\"version\":\"1.0\"}"

== system MCU_Stateflow_Analog/测试/Task_2ms1/Arbitration/Initial ==
  note: WorkCmd初始化
  note: 在POWERON、STANDBY和FAULT模式下ModeSelect选择为cNoneMode
  Action Port : ActionPort
  Constant : Constant  Value=0  OutDataTypeStr=single
  Constant1 : Constant  Value=cNoneMode  VectorParams1D=off  OutDataTypeStr=uint16
  Constant2 : Constant  Value=0  OutDataTypeStr=uint16
  Constant3 : Constant  Value=cNoneMode  VectorParams1D=off  OutDataTypeStr=uint16
  WorkState_ModeSelect : Outport
  WorkCmd_RunCmd : Outport  Port=2
  WorkCmd_DischargeCmd : Outport  Port=3
  WorkCmd_TorqueCmd : Outport  Port=4
  WorkCmd_ModeCmd : Outport  Port=5
  WorkCmd_CurrentCmd : Outport  Port=6
  WorkCmd_FreqCmd : Outport  Port=7
  WorkCmd_IsdCmd : Outport  Port=8
  WorkCmd_IsqCmd : Outport  Port=9
  WorkCmd_SpeedCmd : Outport  Port=10
  WorkCmd_ThetaCmd : Outport  Port=11
  wires:
  Constant/1 -> WorkCmd_TorqueCmd/1, WorkCmd_CurrentCmd/1, WorkCmd_FreqCmd/1, WorkCmd_ThetaCmd/1, WorkCmd_SpeedCmd/1, WorkCmd_IsqCmd/1, WorkCmd_IsdCmd/1
  Constant1/1 -> WorkState_ModeSelect/1
  Constant2/1 -> WorkCmd_RunCmd/1, WorkCmd_DischargeCmd/1
  Constant3/1 -> WorkCmd_ModeCmd/1

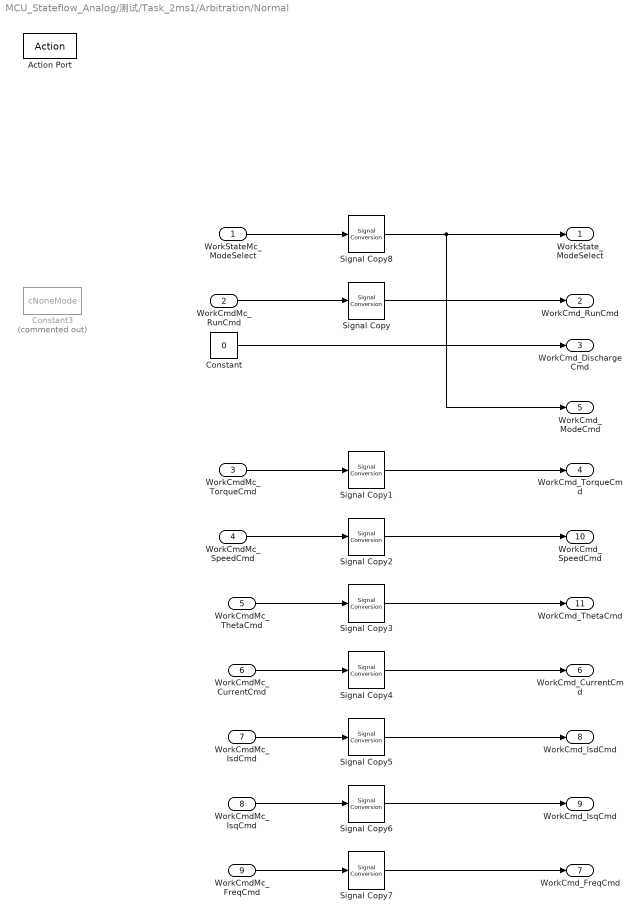
== system MCU_Stateflow_Analog/测试/Task_2ms1/Arbitration/Normal ==
  WorkStateMc_ModeSelect : Inport
  WorkCmdMc_RunCmd : Inport  Port=2
  WorkCmdMc_TorqueCmd : Inport  Port=3
  WorkCmdMc_SpeedCmd : Inport  Port=4
  WorkCmdMc_ThetaCmd : Inport  Port=5
  WorkCmdMc_CurrentCmd : Inport  Port=6
  WorkCmdMc_IsdCmd : Inport  Port=7
  WorkCmdMc_IsqCmd : Inport  Port=8
  WorkCmdMc_FreqCmd : Inport  Port=9
  Action Port : ActionPort
  Constant : Constant  Value=0  OutDataTypeStr=uint16
  Constant3 : Constant  Commented=on  Value=cNoneMode  VectorParams1D=off  OutDataTypeStr=uint16
  Signal Copy{,1..8} (9 alike) : SignalConversion  OverrideOpt=off
  WorkState_ModeSelect : Outport
  WorkCmd_RunCmd : Outport  Port=2
  WorkCmd_DischargeCmd : Outport  Port=3
  WorkCmd_TorqueCmd : Outport  Port=4
  WorkCmd_ModeCmd : Outport  Port=5
  WorkCmd_CurrentCmd : Outport  Port=6
  WorkCmd_FreqCmd : Outport  Port=7
  WorkCmd_IsdCmd : Outport  Port=8
  WorkCmd_IsqCmd : Outport  Port=9
  WorkCmd_SpeedCmd : Outport  Port=10
  WorkCmd_ThetaCmd : Outport  Port=11
  wires:
  WorkCmdMc_RunCmd/1 -> Signal Copy/1
  WorkCmdMc_TorqueCmd/1 -> Signal Copy1/1
  WorkCmdMc_SpeedCmd/1 -> Signal Copy2/1
  WorkCmdMc_ThetaCmd/1 -> Signal Copy3/1
  WorkCmdMc_CurrentCmd/1 -> Signal Copy4/1
  WorkCmdMc_IsdCmd/1 -> Signal Copy5/1
  WorkCmdMc_IsqCmd/1 -> Signal Copy6/1
  WorkCmdMc_FreqCmd/1 -> Signal Copy7/1
  WorkStateMc_ModeSelect/1 -> Signal Copy8/1
  Signal Copy8/1 -> WorkCmd_ModeCmd/1, WorkState_ModeSelect/1
  Signal Copy/1 -> WorkCmd_RunCmd/1
  Signal Copy1/1 -> WorkCmd_TorqueCmd/1
  Signal Copy2/1 -> WorkCmd_SpeedCmd/1
  Signal Copy3/1 -> WorkCmd_ThetaCmd/1
  Signal Copy4/1 -> WorkCmd_CurrentCmd/1
  Signal Copy5/1 -> WorkCmd_IsdCmd/1
  Signal Copy6/1 -> WorkCmd_IsqCmd/1
  Signal Copy7/1 -> WorkCmd_FreqCmd/1
  Constant/1 -> WorkCmd_DischargeCmd/1

== system MCU_Stateflow_Analog/测试/Task_2ms2/Arbitration/Initial ==
  note: WorkCmd初始化
  note: 在POWERON、STANDBY和FAULT模式下ModeSelect选择为cNoneMode
  Action Port : ActionPort
  Constant : Constant  Value=0  OutDataTypeStr=single
  Constant1 : Constant  Value=cNoneMode  VectorParams1D=off  OutDataTypeStr=uint16
  Constant2 : Constant  Value=0  OutDataTypeStr=uint16
  Constant3 : Constant  Value=cNoneMode  VectorParams1D=off  OutDataTypeStr=uint16
  WorkState_ModeSelect : Outport
  WorkCmd_RunCmd : Outport  Port=2
  WorkCmd_DischargeCmd : Outport  Port=3
  WorkCmd_TorqueCmd : Outport  Port=4
  WorkCmd_ModeCmd : Outport  Port=5
  WorkCmd_CurrentCmd : Outport  Port=6
  WorkCmd_FreqCmd : Outport  Port=7
  WorkCmd_IsdCmd : Outport  Port=8
  WorkCmd_IsqCmd : Outport  Port=9
  WorkCmd_SpeedCmd : Outport  Port=10
  WorkCmd_ThetaCmd : Outport  Port=11
  wires:
  Constant/1 -> WorkCmd_TorqueCmd/1, WorkCmd_CurrentCmd/1, WorkCmd_FreqCmd/1, WorkCmd_ThetaCmd/1, WorkCmd_SpeedCmd/1, WorkCmd_IsqCmd/1, WorkCmd_IsdCmd/1
  Constant1/1 -> WorkState_ModeSelect/1
  Constant2/1 -> WorkCmd_RunCmd/1, WorkCmd_DischargeCmd/1
  Constant3/1 -> WorkCmd_ModeCmd/1

== system MCU_Stateflow_Analog/测试/Task_2ms2/Arbitration/Normal ==
  WorkStateMc_ModeSelect : Inport
  WorkCmdMc_RunCmd : Inport  Port=2
  WorkCmdMc_TorqueCmd : Inport  Port=3
  WorkCmdMc_SpeedCmd : Inport  Port=4
  WorkCmdMc_ThetaCmd : Inport  Port=5
  WorkCmdMc_CurrentCmd : Inport  Port=6
  WorkCmdMc_IsdCmd : Inport  Port=7
  WorkCmdMc_IsqCmd : Inport  Port=8
  WorkCmdMc_FreqCmd : Inport  Port=9
  Action Port : ActionPort
  Constant : Constant  Value=0  OutDataTypeStr=uint16
  Constant3 : Constant  Commented=on  Value=cNoneMode  VectorParams1D=off  OutDataTypeStr=uint16
  Signal Copy{,1..8} (9 alike) : SignalConversion  OverrideOpt=off
  WorkState_ModeSelect : Outport
  WorkCmd_RunCmd : Outport  Port=2
  WorkCmd_DischargeCmd : Outport  Port=3
  WorkCmd_TorqueCmd : Outport  Port=4
  WorkCmd_ModeCmd : Outport  Port=5
  WorkCmd_CurrentCmd : Outport  Port=6
  WorkCmd_FreqCmd : Outport  Port=7
  WorkCmd_IsdCmd : Outport  Port=8
  WorkCmd_IsqCmd : Outport  Port=9
  WorkCmd_SpeedCmd : Outport  Port=10
  WorkCmd_ThetaCmd : Outport  Port=11
  wires:
  WorkCmdMc_RunCmd/1 -> Signal Copy/1
  WorkCmdMc_TorqueCmd/1 -> Signal Copy1/1
  WorkCmdMc_SpeedCmd/1 -> Signal Copy2/1
  WorkCmdMc_ThetaCmd/1 -> Signal Copy3/1
  WorkCmdMc_CurrentCmd/1 -> Signal Copy4/1
  WorkCmdMc_IsdCmd/1 -> Signal Copy5/1
  WorkCmdMc_IsqCmd/1 -> Signal Copy6/1
  WorkCmdMc_FreqCmd/1 -> Signal Copy7/1
  WorkStateMc_ModeSelect/1 -> Signal Copy8/1
  Signal Copy8/1 -> WorkCmd_ModeCmd/1, WorkState_ModeSelect/1
  Signal Copy/1 -> WorkCmd_RunCmd/1
  Signal Copy1/1 -> WorkCmd_TorqueCmd/1
  Signal Copy2/1 -> WorkCmd_SpeedCmd/1
  Signal Copy3/1 -> WorkCmd_ThetaCmd/1
  Signal Copy4/1 -> WorkCmd_CurrentCmd/1
  Signal Copy5/1 -> WorkCmd_IsdCmd/1
  Signal Copy6/1 -> WorkCmd_IsqCmd/1
  Signal Copy7/1 -> WorkCmd_FreqCmd/1
  Constant/1 -> WorkCmd_DischargeCmd/1

== stateflow chart MCU_Stateflow_Analog/Task_2ms/草稿/MotorState4 ==
  state PowerOn
    %包括Sensor_Self_Check和Ctrl_Reset
    WorkState_WorkState = POWER_ON
  state Fault
    %WorkState_WorkState = FAULT;
    %{
    WorkState_WorkState = FAULT;
    WorkCmd_RunCmd = WorkCmdMc_RunCmd;
    WorkCmd_DischargeCmd = 0;
    WorkCmd_ModeCmd = cNoneMode;
    WorkCmd_TorqueCmd = 0;
    WorkCmd_SpeedCmd = 0;
    WorkCmd_CurrentCmd = 0;
    WorkCmd_ThetaCmd = 0;
    WorkCmd_IsdCmd = 0;
    WorkCmd_IsqCmd = 0;
    WorkCmd_FreqCmd = 0;
    %}
  state StandBy
    WorkState_WorkState = STANDBY;
  state Working
    WorkState_WorkState = WORKING;
  (default) -> PowerOn
  PowerOn -> (junction 21) : [SelfCheck_OverFlg == 1]
  (junction 13) -> Fault : {WorkState_WorkState = FAULT;
      | WorkState_WorkStateBefore = POWER_ON;
      | WorkState_ModeSelect = cNoneMode;}
  (junction 21) -> (junction 13) [order 1] : [ClosePWMFlag == 1]
  (junction 21) -> StandBy [order 2] : {
      | WorkState_WorkState = STANDBY;
      | WorkState_WorkStateBefore = POWER_ON;
      | WorkState_ModeSelect = cNoneMode;}
  StandBy -> (junction 26) [order 1] : [ClosePWMFlag ==1]
  (junction 26) -> Fault : {WorkState_WorkState = FAULT;
      | WorkState_WorkStateBefore = STANDBY;
      | WorkState_ModeSelect = cNoneMode}
  Fault -> (junction 47) : [ClosePWMFlag ==0]
  (junction 47) -> StandBy : {WorkState_WorkState = STANDBY;
      | WorkState_WorkStateBefore = FAULT;
      | WorkState_ModeSelect = cNoneMode}
  StandBy -> (junction 30) [order 2] : [(WorkCmdSource_ModeCmd ~=cNoneMode & WorkCmdSource_RunCmd==true &Precharge_PrechargeOver==true) ||(WorkCmdSource_ModeCmd ==cSingleBoardMode)]
  (junction 72) -> StandBy : {WorkState_WorkState = STANDBY;
      | WorkState_WorkStateBefore = POWER_ON;
      | WorkState_ModeSelect = cNoneMode;}
  (junction 30) -> Working : {WorkState_WorkState =WORKING;
      | WorkState_WorkStateBefore = STANDBY;}
  Working -> (junction 72) [order 2] : [(WorkCmdSource_RunCmd ==false & WorkState_ModeSelect ~= cSingleBoardMode) || (WorkState_ModeSelect == cNoneMode)]
  (junction 43) -> Fault : {WorkState_WorkState = FAULT;
      | WorkState_WorkStateBefore = WORKING;
      | WorkState_ModeSelect = cNoneMode;}
  Working -> (junction 43) [order 1] : [ClosePWMFlag==1]
  data: SelfCheck_OverFlg input; POWER_ON parameter; ClosePWMFlag input; FAULT parameter; WorkState_WorkState output; WorkState_WorkStateBefore output; cNoneMode parameter; WorkState_ModeSelect output; STANDBY parameter; cSingleBoardMode parameter; WorkCmdSource_RunCmd input; WorkCmdSource_ModeCmd input; Precharge_PrechargeOver input; WORKING parameter

== stateflow chart MCU_Stateflow_Analog/测试/Task_2ms1/MotorState ==
  state PowerOn
    %包括Sensor_Self_Check和Ctrl_Reset
    WorkState_WorkState = POWER_ON;
  state Fault
    %WorkState_WorkState = FAULT;
    %{
    WorkState_WorkState = FAULT;
    WorkCmd_RunCmd = WorkCmdMc_RunCmd;
    WorkCmd_DischargeCmd = 0;
    WorkCmd_ModeCmd = cNoneMode;
    WorkCmd_TorqueCmd = 0;
    WorkCmd_SpeedCmd = 0;
    WorkCmd_CurrentCmd = 0;
    WorkCmd_ThetaCmd = 0;
    WorkCmd_IsdCmd = 0;
    WorkCmd_IsqCmd = 0;
    WorkCmd_FreqCmd = 0;
    %}
  state StandBy
    WorkState_WorkState = STANDBY;
  state Working
    WorkState_WorkState = WORKING;
  (default) -> PowerOn
  PowerOn -> (junction 21) : [SelfCheck_OverFlg == 1]
  (junction 13) -> Fault : {
      | WorkState_WorkState = FAULT;
      | WorkState_WorkStateBefore = POWER_ON;
      | %WorkState_ModeSelect = cNoneMode;
      | }
  (junction 21) -> (junction 13) [order 1] : [ClosePWMFlag == 1]
  (junction 21) -> StandBy [order 2] : {
      | WorkState_WorkState = STANDBY;
      | WorkState_WorkStateBefore = POWER_ON;
      | %WorkState_ModeSelect = cNoneMode;
      | }
  StandBy -> (junction 26) [order 1] : [ClosePWMFlag ==1]
  (junction 26) -> Fault : {
      | WorkState_WorkState = FAULT;
      | WorkState_WorkStateBefore = STANDBY;
      | %WorkState_ModeSelect = cNoneMode
      | }
  Fault -> (junction 47) : [ClosePWMFlag ==0]
  (junction 47) -> StandBy : {
      | WorkState_WorkState = STANDBY;
      | WorkState_WorkStateBefore = FAULT;
      | %WorkState_ModeSelect = cNoneMode
      | }
  StandBy -> (junction 30) [order 2] : [(WorkCmdSource_ModeCmd ~=cNoneMode & WorkCmdSource_RunCmd==true &Precharge_PrechargeOver==true) ||(WorkCmdSource_ModeCmd ==cSingleBoardMode)]
  (junction 72) -> StandBy : {
      | WorkState_WorkState = STANDBY;
      | WorkState_WorkStateBefore = POWER_ON;
      | %WorkState_ModeSelect = cNoneMode;
      | }
  (junction 30) -> Working : {WorkState_WorkState =WORKING;
      | WorkState_WorkStateBefore = STANDBY;}
  Working -> (junction 72) [order 2] : %[(WorkCmdSource_RunCmd ==false & WorkState_ModeSelect ~= cSingleBoardMode) || (WorkState_ModeSelect == cNoneMode)]
      | [(WorkCmdSource_RunCmd ==false & WorkStateMc_ModeSelect ~= cSingleBoardMode) || (WorkStateMc_ModeSelect == cNoneMode)]
  (junction 43) -> Fault : {WorkState_WorkState = FAULT;
      | WorkState_WorkStateBefore = WORKING;
      | %WorkState_ModeSelect = cNoneMode;
      | }
  Working -> (junction 43) [order 1] : [ClosePWMFlag==1]
  data: SelfCheck_OverFlg input; POWER_ON parameter; ClosePWMFlag input; FAULT parameter; WorkState_WorkState output; WorkState_WorkStateBefore output; cNoneMode parameter; STANDBY parameter; cSingleBoardMode parameter; WorkCmdSource_RunCmd input; WorkCmdSource_ModeCmd input; Precharge_PrechargeOver input; WORKING parameter; WorkStateMc_ModeSelect input
